simulink model "chap5_5sim"  (Simulink 8.3)
settings: Solver=ode45  StartTime=0.0  StopTime=5  FixedStep=0.001  RelTol=1e-3
settings Model: Creator=ljk  LastModifiedBy=Prof_Liu  ExtModeTrigMode=oneshot  ExtModeArmWhenConnect=off
settings DataIOCC: LimitDataPoints=off  SignalLoggingName=sigsOut
settings OptimizationCC: BooleanDataType=off  ExpressionDepthLimit=2147483647
settings DebuggingCC: SaveWithParameterizedLinksMsg=none  SignalResolutionControl=TryResolveAllWithWarning  SolverPrmCheckMsg=none  MultiTaskDSMMsg=warning  MultiTaskCondExecSysMsg=none  FcnCallInpInsideContextMsg=UseLocalSettings
settings HardwareCC: TargetUnknown=on
settings RTWCC: IncludeERTFirstTime=on

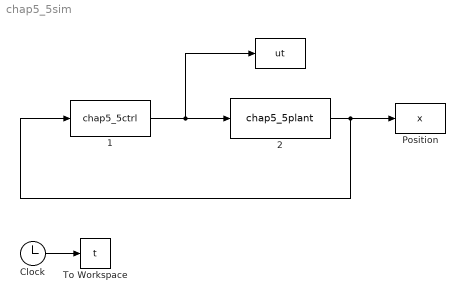
== system chap5_5sim ==
  "  " : ToWorkspace  VariableName=ut  SampleTime=-1
  "  1" : S-Function  FunctionName=chap5_5ctrl  EnableBusSupport=off
  "  2" : S-Function  FunctionName=chap5_5plant  EnableBusSupport=off
  Clock : Clock
  Position : ToWorkspace  VariableName=x  SampleTime=-1
  To Workspace : ToWorkspace  VariableName=t  SampleTime=-1
  wires:
  "  1"/1 -> "  2"/1, "  "/1
  "  2"/1 -> "  1"/1, Position/1
  Clock/1 -> To Workspace/1
